simulink model "gm_wlanhdlTimeAndFrequencySynchronization"  (R2025a)
settings: Solver=FixedStepDiscrete  StartTime=0.0  StopTime=stopTime  RelTol=1e-3
InitFcn:
  | wlanFrontEndInit;
undefined symbols (not defined in the file or in its folder): a, b, c, Hd, wlanConfig
libraries: simulink x95, hdlsllib x16, hdlmdlgenlib x12, dspsrcs4 x3, dspsigops x3, dsphdlsigops2 x2, dsphdlfiltering2 x2
(part 6 of 11)

== system gm_wlanhdlTimeAndFrequencySynchronization/WLANTimeAndFrequencySynchronization/Coarse CFO Estimation and Correction/Coarse CFO Estimation/Iteration2 ==
  xin : Inport  OutDataTypeStr=fixdt(1, 32, 19)  SampleTime=6.25e-09
  yin : Inport  Port=2  OutDataTypeStr=fixdt(1, 32, 19)  SampleTime=6.25e-09
  zin : Inport  Port=3  OutDataTypeStr=fixdt(1, 34, 33)  SampleTime=6.25e-09
  lut_value : Inport  Port=4  OutDataTypeStr=fixdt(0, 31, 33)  SampleTime=6.25e-09
  idx : Inport  Port=5  OutDataTypeStr=fixdt(0, 6, 0)  SampleTime=6.25e-09
  MuxX : Switch  Criteria=u2 ~= 0  Threshold="fi(0,0,1,0,\"hex\",\"0\")"  OutDataTypeStr=fixdt(1, 32, 19)  SampleTime=6.25e-09  SaturateOnIntegerOverflow=off  InputSameDT=off
  MuxY : Switch  Criteria=u2 ~= 0  Threshold="fi(0,0,1,0,\"hex\",\"0\")"  OutDataTypeStr=fixdt(1, 32, 19)  SampleTime=6.25e-09  SaturateOnIntegerOverflow=off  InputSameDT=off
  MuxZ : Switch  Criteria=u2 ~= 0  Threshold="fi(0,0,1,0,\"hex\",\"0\")"  OutDataTypeStr=fixdt(1, 34, 33)  SampleTime=6.25e-09  SaturateOnIntegerOverflow=off  InputSameDT=off
  XAdder : Sum  OutDataTypeStr=fixdt(1, 32, 19)  SampleTime=6.25e-09
  XSubtractor : Sum  Inputs=+-  OutDataTypeStr=fixdt(1, 32, 19)  AccumDataTypeStr=fixdt(1, 32, 19)  SampleTime=6.25e-09
  YAdder : Sum  OutDataTypeStr=fixdt(1, 32, 19)  SampleTime=6.25e-09
  YSub : Sum  Inputs=+-  OutDataTypeStr=fixdt(1, 32, 19)  AccumDataTypeStr=fixdt(1, 32, 19)  SampleTime=6.25e-09
  ZAdder : Sum  OutDataTypeStr=fixdt(1, 34, 33)  SampleTime=6.25e-09
  ZSub : Sum  Inputs=+-  OutDataTypeStr=fixdt(1, 34, 33)  AccumDataTypeStr=fixdt(1, 34, 33)  SampleTime=6.25e-09
  compare : simulink/Logic and Bit Operations/Compare To Constant  relop=<  const=double(0)  OutDataTypeStr=boolean
  dynamic_shift : ArithShift  BitShiftNumberSource=Input port  BitShiftDirection=Right
      settings: InputPortMap=u0,p1
  dynamic_shift1 : ArithShift  BitShiftNumberSource=Input port  BitShiftDirection=Right
      settings: InputPortMap=u0,p1
  rd_{0..9} (10 alike) : Delay  DelayLength=double(1)  InitialCondition=0  SampleTime=6.25e-09
  xout : Outport  OutDataTypeStr=fixdt(1, 32, 19)  SampleTime=6.25e-09
  yout : Outport  Port=2  OutDataTypeStr=fixdt(1, 32, 19)  SampleTime=6.25e-09
  zout : Outport  Port=3  OutDataTypeStr=fixdt(1, 34, 33)  SampleTime=6.25e-09
  wires:
  MuxZ/1 -> zout/1
  rd_6/1 -> MuxY/3
  rd_9/1 -> MuxZ/3
  rd_2/1 -> MuxX/1
  rd_5/1 -> MuxY/1
  YSub/1 -> rd_6/1
  ZSub/1 -> rd_8/1
  xin/1 -> rd_0/1
  YAdder/1 -> rd_5/1
  lut_value/1 -> ZAdder/2, ZSub/2
  yin/1 -> rd_1/1
  rd_0/1 -> dynamic_shift/1, XAdder/1, XSubtractor/1
  MuxX/1 -> xout/1
  zin/1 -> rd_7/1
  MuxY/1 -> yout/1
  rd_1/1 -> compare/1, dynamic_shift1/1, YAdder/1, YSub/1
  idx/1 -> dynamic_shift1/2, dynamic_shift/2
  dynamic_shift1/1 -> XAdder/2, XSubtractor/2
  rd_3/1 -> MuxX/2, MuxY/2, MuxZ/2
  rd_7/1 -> ZSub/1, ZAdder/1
  rd_4/1 -> MuxX/3
  XAdder/1 -> rd_4/1
  compare/1 -> rd_3/1
  rd_8/1 -> MuxZ/1
  dynamic_shift/1 -> YSub/2, YAdder/2
  ZAdder/1 -> rd_9/1
  XSubtractor/1 -> rd_2/1

== system gm_wlanhdlTimeAndFrequencySynchronization/WLANTimeAndFrequencySynchronization/Coarse CFO Estimation and Correction/Coarse CFO Estimation/Iteration20 ==
  xin : Inport  OutDataTypeStr=fixdt(1, 32, 19)  SampleTime=6.25e-09
  yin : Inport  Port=2  OutDataTypeStr=fixdt(1, 32, 19)  SampleTime=6.25e-09
  zin : Inport  Port=3  OutDataTypeStr=fixdt(1, 34, 33)  SampleTime=6.25e-09
  lut_value : Inport  Port=4  OutDataTypeStr=fixdt(0, 31, 33)  SampleTime=6.25e-09
  idx : Inport  Port=5  OutDataTypeStr=fixdt(0, 6, 0)  SampleTime=6.25e-09
  MuxX : Switch  Criteria=u2 ~= 0  Threshold="fi(0,0,1,0,\"hex\",\"0\")"  OutDataTypeStr=fixdt(1, 32, 19)  SampleTime=6.25e-09  SaturateOnIntegerOverflow=off  InputSameDT=off
  MuxY : Switch  Criteria=u2 ~= 0  Threshold="fi(0,0,1,0,\"hex\",\"0\")"  OutDataTypeStr=fixdt(1, 32, 19)  SampleTime=6.25e-09  SaturateOnIntegerOverflow=off  InputSameDT=off
  MuxZ : Switch  Criteria=u2 ~= 0  Threshold="fi(0,0,1,0,\"hex\",\"0\")"  OutDataTypeStr=fixdt(1, 34, 33)  SampleTime=6.25e-09  SaturateOnIntegerOverflow=off  InputSameDT=off
  XAdder : Sum  OutDataTypeStr=fixdt(1, 32, 19)  SampleTime=6.25e-09
  XSubtractor : Sum  Inputs=+-  OutDataTypeStr=fixdt(1, 32, 19)  AccumDataTypeStr=fixdt(1, 32, 19)  SampleTime=6.25e-09
  YAdder : Sum  OutDataTypeStr=fixdt(1, 32, 19)  SampleTime=6.25e-09
  YSub : Sum  Inputs=+-  OutDataTypeStr=fixdt(1, 32, 19)  AccumDataTypeStr=fixdt(1, 32, 19)  SampleTime=6.25e-09
  ZAdder : Sum  OutDataTypeStr=fixdt(1, 34, 33)  SampleTime=6.25e-09
  ZSub : Sum  Inputs=+-  OutDataTypeStr=fixdt(1, 34, 33)  AccumDataTypeStr=fixdt(1, 34, 33)  SampleTime=6.25e-09
  compare : simulink/Logic and Bit Operations/Compare To Constant  relop=<  const=double(0)  OutDataTypeStr=boolean
  dynamic_shift : ArithShift  BitShiftNumberSource=Input port  BitShiftDirection=Right
      settings: InputPortMap=u0,p1
  dynamic_shift1 : ArithShift  BitShiftNumberSource=Input port  BitShiftDirection=Right
      settings: InputPortMap=u0,p1
  rd_{0..9} (10 alike) : Delay  DelayLength=double(1)  InitialCondition=0  SampleTime=6.25e-09
  xout : Outport  OutDataTypeStr=fixdt(1, 32, 19)  SampleTime=6.25e-09
  yout : Outport  Port=2  OutDataTypeStr=fixdt(1, 32, 19)  SampleTime=6.25e-09
  zout : Outport  Port=3  OutDataTypeStr=fixdt(1, 34, 33)  SampleTime=6.25e-09
  wires:
  MuxY/1 -> yout/1
  rd_4/1 -> MuxX/3
  rd_9/1 -> MuxZ/3
  rd_6/1 -> MuxY/3
  XAdder/1 -> rd_4/1
  ZAdder/1 -> rd_9/1
  rd_3/1 -> MuxX/2, MuxY/2, MuxZ/2
  yin/1 -> rd_1/1
  rd_8/1 -> MuxZ/1
  xin/1 -> rd_0/1
  MuxX/1 -> xout/1
  ZSub/1 -> rd_8/1
  zin/1 -> rd_7/1
  MuxZ/1 -> zout/1
  idx/1 -> dynamic_shift1/2, dynamic_shift/2
  rd_0/1 -> dynamic_shift/1, XSubtractor/1, XAdder/1
  rd_1/1 -> compare/1, dynamic_shift1/1, YAdder/1, YSub/1
  YSub/1 -> rd_6/1
  rd_2/1 -> MuxX/1
  dynamic_shift/1 -> YSub/2, YAdder/2
  XSubtractor/1 -> rd_2/1
  rd_7/1 -> ZSub/1, ZAdder/1
  rd_5/1 -> MuxY/1
  lut_value/1 -> ZAdder/2, ZSub/2
  dynamic_shift1/1 -> XAdder/2, XSubtractor/2
  compare/1 -> rd_3/1
  YAdder/1 -> rd_5/1

== system gm_wlanhdlTimeAndFrequencySynchronization/WLANTimeAndFrequencySynchronization/Coarse CFO Estimation and Correction/Coarse CFO Estimation/Iteration21 ==
  xin : Inport  OutDataTypeStr=fixdt(1, 32, 19)  SampleTime=6.25e-09
  yin : Inport  Port=2  OutDataTypeStr=fixdt(1, 32, 19)  SampleTime=6.25e-09
  zin : Inport  Port=3  OutDataTypeStr=fixdt(1, 34, 33)  SampleTime=6.25e-09
  lut_value : Inport  Port=4  OutDataTypeStr=fixdt(0, 31, 33)  SampleTime=6.25e-09
  idx : Inport  Port=5  OutDataTypeStr=fixdt(0, 6, 0)  SampleTime=6.25e-09
  MuxX : Switch  Criteria=u2 ~= 0  Threshold="fi(0,0,1,0,\"hex\",\"0\")"  OutDataTypeStr=fixdt(1, 32, 19)  SampleTime=6.25e-09  SaturateOnIntegerOverflow=off  InputSameDT=off
  MuxY : Switch  Criteria=u2 ~= 0  Threshold="fi(0,0,1,0,\"hex\",\"0\")"  OutDataTypeStr=fixdt(1, 32, 19)  SampleTime=6.25e-09  SaturateOnIntegerOverflow=off  InputSameDT=off
  MuxZ : Switch  Criteria=u2 ~= 0  Threshold="fi(0,0,1,0,\"hex\",\"0\")"  OutDataTypeStr=fixdt(1, 34, 33)  SampleTime=6.25e-09  SaturateOnIntegerOverflow=off  InputSameDT=off
  XAdder : Sum  OutDataTypeStr=fixdt(1, 32, 19)  SampleTime=6.25e-09
  XSubtractor : Sum  Inputs=+-  OutDataTypeStr=fixdt(1, 32, 19)  AccumDataTypeStr=fixdt(1, 32, 19)  SampleTime=6.25e-09
  YAdder : Sum  OutDataTypeStr=fixdt(1, 32, 19)  SampleTime=6.25e-09
  YSub : Sum  Inputs=+-  OutDataTypeStr=fixdt(1, 32, 19)  AccumDataTypeStr=fixdt(1, 32, 19)  SampleTime=6.25e-09
  ZAdder : Sum  OutDataTypeStr=fixdt(1, 34, 33)  SampleTime=6.25e-09
  ZSub : Sum  Inputs=+-  OutDataTypeStr=fixdt(1, 34, 33)  AccumDataTypeStr=fixdt(1, 34, 33)  SampleTime=6.25e-09
  compare : simulink/Logic and Bit Operations/Compare To Constant  relop=<  const=double(0)  OutDataTypeStr=boolean
  dynamic_shift : ArithShift  BitShiftNumberSource=Input port  BitShiftDirection=Right
      settings: InputPortMap=u0,p1
  dynamic_shift1 : ArithShift  BitShiftNumberSource=Input port  BitShiftDirection=Right
      settings: InputPortMap=u0,p1
  rd_{0..9} (10 alike) : Delay  DelayLength=double(1)  InitialCondition=0  SampleTime=6.25e-09
  xout : Outport  OutDataTypeStr=fixdt(1, 32, 19)  SampleTime=6.25e-09
  yout : Outport  Port=2  OutDataTypeStr=fixdt(1, 32, 19)  SampleTime=6.25e-09
  zout : Outport  Port=3  OutDataTypeStr=fixdt(1, 34, 33)  SampleTime=6.25e-09
  wires:
  MuxY/1 -> yout/1
  rd_2/1 -> MuxX/1
  rd_5/1 -> MuxY/1
  XAdder/1 -> rd_4/1
  MuxX/1 -> xout/1
  XSubtractor/1 -> rd_2/1
  rd_4/1 -> MuxX/3
  rd_8/1 -> MuxZ/1
  ZAdder/1 -> rd_9/1
  rd_3/1 -> MuxX/2, MuxY/2, MuxZ/2
  ZSub/1 -> rd_8/1
  yin/1 -> rd_1/1
  xin/1 -> rd_0/1
  rd_1/1 -> compare/1, dynamic_shift1/1, YAdder/1, YSub/1
  YAdder/1 -> rd_5/1
  dynamic_shift/1 -> YAdder/2, YSub/2
  MuxZ/1 -> zout/1
  rd_0/1 -> dynamic_shift/1, XAdder/1, XSubtractor/1
  idx/1 -> dynamic_shift/2, dynamic_shift1/2
  dynamic_shift1/1 -> XSubtractor/2, XAdder/2
  rd_6/1 -> MuxY/3
  rd_7/1 -> ZSub/1, ZAdder/1
  lut_value/1 -> ZSub/2, ZAdder/2
  compare/1 -> rd_3/1
  rd_9/1 -> MuxZ/3
  zin/1 -> rd_7/1
  YSub/1 -> rd_6/1

== system gm_wlanhdlTimeAndFrequencySynchronization/WLANTimeAndFrequencySynchronization/Coarse CFO Estimation and Correction/Coarse CFO Estimation/Iteration22 ==
  xin : Inport  OutDataTypeStr=fixdt(1, 32, 19)  SampleTime=6.25e-09
  yin : Inport  Port=2  OutDataTypeStr=fixdt(1, 32, 19)  SampleTime=6.25e-09
  zin : Inport  Port=3  OutDataTypeStr=fixdt(1, 34, 33)  SampleTime=6.25e-09
  lut_value : Inport  Port=4  OutDataTypeStr=fixdt(0, 31, 33)  SampleTime=6.25e-09
  idx : Inport  Port=5  OutDataTypeStr=fixdt(0, 6, 0)  SampleTime=6.25e-09
  MuxX : Switch  Criteria=u2 ~= 0  Threshold="fi(0,0,1,0,\"hex\",\"0\")"  OutDataTypeStr=fixdt(1, 32, 19)  SampleTime=6.25e-09  SaturateOnIntegerOverflow=off  InputSameDT=off
  MuxY : Switch  Criteria=u2 ~= 0  Threshold="fi(0,0,1,0,\"hex\",\"0\")"  OutDataTypeStr=fixdt(1, 32, 19)  SampleTime=6.25e-09  SaturateOnIntegerOverflow=off  InputSameDT=off
  MuxZ : Switch  Criteria=u2 ~= 0  Threshold="fi(0,0,1,0,\"hex\",\"0\")"  OutDataTypeStr=fixdt(1, 34, 33)  SampleTime=6.25e-09  SaturateOnIntegerOverflow=off  InputSameDT=off
  XAdder : Sum  OutDataTypeStr=fixdt(1, 32, 19)  SampleTime=6.25e-09
  XSubtractor : Sum  Inputs=+-  OutDataTypeStr=fixdt(1, 32, 19)  AccumDataTypeStr=fixdt(1, 32, 19)  SampleTime=6.25e-09
  YAdder : Sum  OutDataTypeStr=fixdt(1, 32, 19)  SampleTime=6.25e-09
  YSub : Sum  Inputs=+-  OutDataTypeStr=fixdt(1, 32, 19)  AccumDataTypeStr=fixdt(1, 32, 19)  SampleTime=6.25e-09
  ZAdder : Sum  OutDataTypeStr=fixdt(1, 34, 33)  SampleTime=6.25e-09
  ZSub : Sum  Inputs=+-  OutDataTypeStr=fixdt(1, 34, 33)  AccumDataTypeStr=fixdt(1, 34, 33)  SampleTime=6.25e-09
  compare : simulink/Logic and Bit Operations/Compare To Constant  relop=<  const=double(0)  OutDataTypeStr=boolean
  dynamic_shift : ArithShift  BitShiftNumberSource=Input port  BitShiftDirection=Right
      settings: InputPortMap=u0,p1
  dynamic_shift1 : ArithShift  BitShiftNumberSource=Input port  BitShiftDirection=Right
      settings: InputPortMap=u0,p1
  rd_{0..9} (10 alike) : Delay  DelayLength=double(1)  InitialCondition=0  SampleTime=6.25e-09
  xout : Outport  OutDataTypeStr=fixdt(1, 32, 19)  SampleTime=6.25e-09
  yout : Outport  Port=2  OutDataTypeStr=fixdt(1, 32, 19)  SampleTime=6.25e-09
  zout : Outport  Port=3  OutDataTypeStr=fixdt(1, 34, 33)  SampleTime=6.25e-09
  wires:
  MuxX/1 -> xout/1
  MuxY/1 -> yout/1
  rd_4/1 -> MuxX/3
  rd_2/1 -> MuxX/1
  rd_3/1 -> MuxX/2, MuxY/2, MuxZ/2
  XAdder/1 -> rd_4/1
  XSubtractor/1 -> rd_2/1
  ZAdder/1 -> rd_9/1
  rd_9/1 -> MuxZ/3
  ZSub/1 -> rd_8/1
  compare/1 -> rd_3/1
  rd_8/1 -> MuxZ/1
  rd_5/1 -> MuxY/1
  yin/1 -> rd_1/1
  rd_1/1 -> compare/1, dynamic_shift1/1, YAdder/1, YSub/1
  dynamic_shift1/1 -> XAdder/2, XSubtractor/2
  zin/1 -> rd_7/1
  MuxZ/1 -> zout/1
  idx/1 -> dynamic_shift1/2, dynamic_shift/2
  YSub/1 -> rd_6/1
  rd_0/1 -> dynamic_shift/1, XSubtractor/1, XAdder/1
  dynamic_shift/1 -> YSub/2, YAdder/2
  rd_7/1 -> ZSub/1, ZAdder/1
  rd_6/1 -> MuxY/3
  lut_value/1 -> ZAdder/2, ZSub/2
  xin/1 -> rd_0/1
  YAdder/1 -> rd_5/1

== system gm_wlanhdlTimeAndFrequencySynchronization/WLANTimeAndFrequencySynchronization/Coarse CFO Estimation and Correction/Coarse CFO Estimation/Iteration23 ==
  xin : Inport  OutDataTypeStr=fixdt(1, 32, 19)  SampleTime=6.25e-09
  yin : Inport  Port=2  OutDataTypeStr=fixdt(1, 32, 19)  SampleTime=6.25e-09
  zin : Inport  Port=3  OutDataTypeStr=fixdt(1, 34, 33)  SampleTime=6.25e-09
  lut_value : Inport  Port=4  OutDataTypeStr=fixdt(0, 31, 33)  SampleTime=6.25e-09
  idx : Inport  Port=5  OutDataTypeStr=fixdt(0, 6, 0)  SampleTime=6.25e-09
  MuxX : Switch  Criteria=u2 ~= 0  Threshold="fi(0,0,1,0,\"hex\",\"0\")"  OutDataTypeStr=fixdt(1, 32, 19)  SampleTime=6.25e-09  SaturateOnIntegerOverflow=off  InputSameDT=off
  MuxY : Switch  Criteria=u2 ~= 0  Threshold="fi(0,0,1,0,\"hex\",\"0\")"  OutDataTypeStr=fixdt(1, 32, 19)  SampleTime=6.25e-09  SaturateOnIntegerOverflow=off  InputSameDT=off
  MuxZ : Switch  Criteria=u2 ~= 0  Threshold="fi(0,0,1,0,\"hex\",\"0\")"  OutDataTypeStr=fixdt(1, 34, 33)  SampleTime=6.25e-09  SaturateOnIntegerOverflow=off  InputSameDT=off
  XAdder : Sum  OutDataTypeStr=fixdt(1, 32, 19)  SampleTime=6.25e-09
  XSubtractor : Sum  Inputs=+-  OutDataTypeStr=fixdt(1, 32, 19)  AccumDataTypeStr=fixdt(1, 32, 19)  SampleTime=6.25e-09
  YAdder : Sum  OutDataTypeStr=fixdt(1, 32, 19)  SampleTime=6.25e-09
  YSub : Sum  Inputs=+-  OutDataTypeStr=fixdt(1, 32, 19)  AccumDataTypeStr=fixdt(1, 32, 19)  SampleTime=6.25e-09
  ZAdder : Sum  OutDataTypeStr=fixdt(1, 34, 33)  SampleTime=6.25e-09
  ZSub : Sum  Inputs=+-  OutDataTypeStr=fixdt(1, 34, 33)  AccumDataTypeStr=fixdt(1, 34, 33)  SampleTime=6.25e-09
  compare : simulink/Logic and Bit Operations/Compare To Constant  relop=<  const=double(0)  OutDataTypeStr=boolean
  dynamic_shift : ArithShift  BitShiftNumberSource=Input port  BitShiftDirection=Right
      settings: InputPortMap=u0,p1
  dynamic_shift1 : ArithShift  BitShiftNumberSource=Input port  BitShiftDirection=Right
      settings: InputPortMap=u0,p1
  rd_{0..9} (10 alike) : Delay  DelayLength=double(1)  InitialCondition=0  SampleTime=6.25e-09
  xout : Outport  OutDataTypeStr=fixdt(1, 32, 19)  SampleTime=6.25e-09
  yout : Outport  Port=2  OutDataTypeStr=fixdt(1, 32, 19)  SampleTime=6.25e-09
  zout : Outport  Port=3  OutDataTypeStr=fixdt(1, 34, 33)  SampleTime=6.25e-09
  wires:
  MuxZ/1 -> zout/1
  rd_3/1 -> MuxX/2, MuxZ/2, MuxY/2
  rd_9/1 -> MuxZ/3
  YAdder/1 -> rd_5/1
  yin/1 -> rd_1/1
  MuxX/1 -> xout/1
  XSubtractor/1 -> rd_2/1
  rd_1/1 -> compare/1, dynamic_shift1/1, YAdder/1, YSub/1
  rd_5/1 -> MuxY/1
  ZSub/1 -> rd_8/1
  MuxY/1 -> yout/1
  XAdder/1 -> rd_4/1
  xin/1 -> rd_0/1
  idx/1 -> dynamic_shift/2, dynamic_shift1/2
  rd_0/1 -> dynamic_shift/1, XAdder/1, XSubtractor/1
  dynamic_shift1/1 -> XSubtractor/2, XAdder/2
  zin/1 -> rd_7/1
  ZAdder/1 -> rd_9/1
  rd_4/1 -> MuxX/3
  rd_6/1 -> MuxY/3
  YSub/1 -> rd_6/1
  rd_7/1 -> ZSub/1, ZAdder/1
  rd_2/1 -> MuxX/1
  dynamic_shift/1 -> YAdder/2, YSub/2
  rd_8/1 -> MuxZ/1
  lut_value/1 -> ZSub/2, ZAdder/2
  compare/1 -> rd_3/1

== system gm_wlanhdlTimeAndFrequencySynchronization/WLANTimeAndFrequencySynchronization/Coarse CFO Estimation and Correction/Coarse CFO Estimation/Iteration24 ==
  xin : Inport  OutDataTypeStr=fixdt(1, 32, 19)  SampleTime=6.25e-09
  yin : Inport  Port=2  OutDataTypeStr=fixdt(1, 32, 19)  SampleTime=6.25e-09
  zin : Inport  Port=3  OutDataTypeStr=fixdt(1, 34, 33)  SampleTime=6.25e-09
  lut_value : Inport  Port=4  OutDataTypeStr=fixdt(0, 31, 33)  SampleTime=6.25e-09
  idx : Inport  Port=5  OutDataTypeStr=fixdt(0, 6, 0)  SampleTime=6.25e-09
  MuxX : Switch  Criteria=u2 ~= 0  Threshold="fi(0,0,1,0,\"hex\",\"0\")"  OutDataTypeStr=fixdt(1, 32, 19)  SampleTime=6.25e-09  SaturateOnIntegerOverflow=off  InputSameDT=off
  MuxY : Switch  Criteria=u2 ~= 0  Threshold="fi(0,0,1,0,\"hex\",\"0\")"  OutDataTypeStr=fixdt(1, 32, 19)  SampleTime=6.25e-09  SaturateOnIntegerOverflow=off  InputSameDT=off
  MuxZ : Switch  Criteria=u2 ~= 0  Threshold="fi(0,0,1,0,\"hex\",\"0\")"  OutDataTypeStr=fixdt(1, 34, 33)  SampleTime=6.25e-09  SaturateOnIntegerOverflow=off  InputSameDT=off
  XAdder : Sum  OutDataTypeStr=fixdt(1, 32, 19)  SampleTime=6.25e-09
  XSubtractor : Sum  Inputs=+-  OutDataTypeStr=fixdt(1, 32, 19)  AccumDataTypeStr=fixdt(1, 32, 19)  SampleTime=6.25e-09
  YAdder : Sum  OutDataTypeStr=fixdt(1, 32, 19)  SampleTime=6.25e-09
  YSub : Sum  Inputs=+-  OutDataTypeStr=fixdt(1, 32, 19)  AccumDataTypeStr=fixdt(1, 32, 19)  SampleTime=6.25e-09
  ZAdder : Sum  OutDataTypeStr=fixdt(1, 34, 33)  SampleTime=6.25e-09
  ZSub : Sum  Inputs=+-  OutDataTypeStr=fixdt(1, 34, 33)  AccumDataTypeStr=fixdt(1, 34, 33)  SampleTime=6.25e-09
  compare : simulink/Logic and Bit Operations/Compare To Constant  relop=<  const=double(0)  OutDataTypeStr=boolean
  dynamic_shift : ArithShift  BitShiftNumberSource=Input port  BitShiftDirection=Right
      settings: InputPortMap=u0,p1
  dynamic_shift1 : ArithShift  BitShiftNumberSource=Input port  BitShiftDirection=Right
      settings: InputPortMap=u0,p1
  rd_{0..9} (10 alike) : Delay  DelayLength=double(1)  InitialCondition=0  SampleTime=6.25e-09
  xout : Outport  OutDataTypeStr=fixdt(1, 32, 19)  SampleTime=6.25e-09
  yout : Outport  Port=2  OutDataTypeStr=fixdt(1, 32, 19)  SampleTime=6.25e-09
  zout : Outport  Port=3  OutDataTypeStr=fixdt(1, 34, 33)  SampleTime=6.25e-09
  wires:
  MuxZ/1 -> zout/1
  rd_2/1 -> MuxX/1
  rd_9/1 -> MuxZ/3
  rd_3/1 -> MuxX/2, MuxY/2, MuxZ/2
  rd_6/1 -> MuxY/3
  MuxY/1 -> yout/1
  rd_8/1 -> MuxZ/1
  XAdder/1 -> rd_4/1
  ZAdder/1 -> rd_9/1
  yin/1 -> rd_1/1
  MuxX/1 -> xout/1
  compare/1 -> rd_3/1
  rd_5/1 -> MuxY/1
  xin/1 -> rd_0/1
  rd_7/1 -> ZSub/1, ZAdder/1
  rd_1/1 -> compare/1, YAdder/1, dynamic_shift1/1, YSub/1
  zin/1 -> rd_7/1
  YSub/1 -> rd_6/1
  idx/1 -> dynamic_shift1/2, dynamic_shift/2
  rd_0/1 -> dynamic_shift/1, XSubtractor/1, XAdder/1
  dynamic_shift/1 -> YSub/2, YAdder/2
  ZSub/1 -> rd_8/1
  dynamic_shift1/1 -> XAdder/2, XSubtractor/2
  rd_4/1 -> MuxX/3
  lut_value/1 -> ZAdder/2, ZSub/2
  XSubtractor/1 -> rd_2/1
  YAdder/1 -> rd_5/1

== system gm_wlanhdlTimeAndFrequencySynchronization/WLANTimeAndFrequencySynchronization/Coarse CFO Estimation and Correction/Coarse CFO Estimation/Iteration25 ==
  xin : Inport  OutDataTypeStr=fixdt(1, 32, 19)  SampleTime=6.25e-09
  yin : Inport  Port=2  OutDataTypeStr=fixdt(1, 32, 19)  SampleTime=6.25e-09
  zin : Inport  Port=3  OutDataTypeStr=fixdt(1, 34, 33)  SampleTime=6.25e-09
  lut_value : Inport  Port=4  OutDataTypeStr=fixdt(0, 31, 33)  SampleTime=6.25e-09
  idx : Inport  Port=5  OutDataTypeStr=fixdt(0, 6, 0)  SampleTime=6.25e-09
  MuxX : Switch  Criteria=u2 ~= 0  Threshold="fi(0,0,1,0,\"hex\",\"0\")"  OutDataTypeStr=fixdt(1, 32, 19)  SampleTime=6.25e-09  SaturateOnIntegerOverflow=off  InputSameDT=off
  MuxY : Switch  Criteria=u2 ~= 0  Threshold="fi(0,0,1,0,\"hex\",\"0\")"  OutDataTypeStr=fixdt(1, 32, 19)  SampleTime=6.25e-09  SaturateOnIntegerOverflow=off  InputSameDT=off
  MuxZ : Switch  Criteria=u2 ~= 0  Threshold="fi(0,0,1,0,\"hex\",\"0\")"  OutDataTypeStr=fixdt(1, 34, 33)  SampleTime=6.25e-09  SaturateOnIntegerOverflow=off  InputSameDT=off
  XAdder : Sum  OutDataTypeStr=fixdt(1, 32, 19)  SampleTime=6.25e-09
  XSubtractor : Sum  Inputs=+-  OutDataTypeStr=fixdt(1, 32, 19)  AccumDataTypeStr=fixdt(1, 32, 19)  SampleTime=6.25e-09
  YAdder : Sum  OutDataTypeStr=fixdt(1, 32, 19)  SampleTime=6.25e-09
  YSub : Sum  Inputs=+-  OutDataTypeStr=fixdt(1, 32, 19)  AccumDataTypeStr=fixdt(1, 32, 19)  SampleTime=6.25e-09
  ZAdder : Sum  OutDataTypeStr=fixdt(1, 34, 33)  SampleTime=6.25e-09
  ZSub : Sum  Inputs=+-  OutDataTypeStr=fixdt(1, 34, 33)  AccumDataTypeStr=fixdt(1, 34, 33)  SampleTime=6.25e-09
  compare : simulink/Logic and Bit Operations/Compare To Constant  relop=<  const=double(0)  OutDataTypeStr=boolean
  dynamic_shift : ArithShift  BitShiftNumberSource=Input port  BitShiftDirection=Right
      settings: InputPortMap=u0,p1
  dynamic_shift1 : ArithShift  BitShiftNumberSource=Input port  BitShiftDirection=Right
      settings: InputPortMap=u0,p1
  rd_{0..9} (10 alike) : Delay  DelayLength=double(1)  InitialCondition=0  SampleTime=6.25e-09
  xout : Outport  OutDataTypeStr=fixdt(1, 32, 19)  SampleTime=6.25e-09
  yout : Outport  Port=2  OutDataTypeStr=fixdt(1, 32, 19)  SampleTime=6.25e-09
  zout : Outport  Port=3  OutDataTypeStr=fixdt(1, 34, 33)  SampleTime=6.25e-09
  wires:
  MuxZ/1 -> zout/1
  rd_2/1 -> MuxX/1
  rd_4/1 -> MuxX/3
  rd_9/1 -> MuxZ/3
  rd_3/1 -> MuxX/2, MuxY/2, MuxZ/2
  rd_8/1 -> MuxZ/1
  rd_6/1 -> MuxY/3
  MuxY/1 -> yout/1
  rd_5/1 -> MuxY/1
  XSubtractor/1 -> rd_2/1
  ZAdder/1 -> rd_9/1
  ZSub/1 -> rd_8/1
  lut_value/1 -> ZSub/2, ZAdder/2
  xin/1 -> rd_0/1
  YAdder/1 -> rd_5/1
  XAdder/1 -> rd_4/1
  rd_1/1 -> compare/1, dynamic_shift1/1, YAdder/1, YSub/1
  yin/1 -> rd_1/1
  zin/1 -> rd_7/1
  idx/1 -> dynamic_shift/2, dynamic_shift1/2
  MuxX/1 -> xout/1
  dynamic_shift/1 -> YAdder/2, YSub/2
  compare/1 -> rd_3/1
  rd_0/1 -> dynamic_shift/1, XSubtractor/1, XAdder/1
  dynamic_shift1/1 -> XSubtractor/2, XAdder/2
  rd_7/1 -> ZSub/1, ZAdder/1
  YSub/1 -> rd_6/1

== system gm_wlanhdlTimeAndFrequencySynchronization/WLANTimeAndFrequencySynchronization/Coarse CFO Estimation and Correction/Coarse CFO Estimation/Iteration26 ==
  xin : Inport  OutDataTypeStr=fixdt(1, 32, 19)  SampleTime=6.25e-09
  yin : Inport  Port=2  OutDataTypeStr=fixdt(1, 32, 19)  SampleTime=6.25e-09
  zin : Inport  Port=3  OutDataTypeStr=fixdt(1, 34, 33)  SampleTime=6.25e-09
  lut_value : Inport  Port=4  OutDataTypeStr=fixdt(0, 31, 33)  SampleTime=6.25e-09
  idx : Inport  Port=5  OutDataTypeStr=fixdt(0, 6, 0)  SampleTime=6.25e-09
  MuxX : Switch  Criteria=u2 ~= 0  Threshold="fi(0,0,1,0,\"hex\",\"0\")"  OutDataTypeStr=fixdt(1, 32, 19)  SampleTime=6.25e-09  SaturateOnIntegerOverflow=off  InputSameDT=off
  MuxY : Switch  Criteria=u2 ~= 0  Threshold="fi(0,0,1,0,\"hex\",\"0\")"  OutDataTypeStr=fixdt(1, 32, 19)  SampleTime=6.25e-09  SaturateOnIntegerOverflow=off  InputSameDT=off
  MuxZ : Switch  Criteria=u2 ~= 0  Threshold="fi(0,0,1,0,\"hex\",\"0\")"  OutDataTypeStr=fixdt(1, 34, 33)  SampleTime=6.25e-09  SaturateOnIntegerOverflow=off  InputSameDT=off
  XAdder : Sum  OutDataTypeStr=fixdt(1, 32, 19)  SampleTime=6.25e-09
  XSubtractor : Sum  Inputs=+-  OutDataTypeStr=fixdt(1, 32, 19)  AccumDataTypeStr=fixdt(1, 32, 19)  SampleTime=6.25e-09
  YAdder : Sum  OutDataTypeStr=fixdt(1, 32, 19)  SampleTime=6.25e-09
  YSub : Sum  Inputs=+-  OutDataTypeStr=fixdt(1, 32, 19)  AccumDataTypeStr=fixdt(1, 32, 19)  SampleTime=6.25e-09
  ZAdder : Sum  OutDataTypeStr=fixdt(1, 34, 33)  SampleTime=6.25e-09
  ZSub : Sum  Inputs=+-  OutDataTypeStr=fixdt(1, 34, 33)  AccumDataTypeStr=fixdt(1, 34, 33)  SampleTime=6.25e-09
  compare : simulink/Logic and Bit Operations/Compare To Constant  relop=<  const=double(0)  OutDataTypeStr=boolean
  dynamic_shift : ArithShift  BitShiftNumberSource=Input port  BitShiftDirection=Right
      settings: InputPortMap=u0,p1
  dynamic_shift1 : ArithShift  BitShiftNumberSource=Input port  BitShiftDirection=Right
      settings: InputPortMap=u0,p1
  rd_{0..9} (10 alike) : Delay  DelayLength=double(1)  InitialCondition=0  SampleTime=6.25e-09
  xout : Outport  OutDataTypeStr=fixdt(1, 32, 19)  SampleTime=6.25e-09
  yout : Outport  Port=2  OutDataTypeStr=fixdt(1, 32, 19)  SampleTime=6.25e-09
  zout : Outport  Port=3  OutDataTypeStr=fixdt(1, 34, 33)  SampleTime=6.25e-09
  wires:
  MuxX/1 -> xout/1
  MuxY/1 -> yout/1
  rd_9/1 -> MuxZ/3
  rd_8/1 -> MuxZ/1
  ZAdder/1 -> rd_9/1
  ZSub/1 -> rd_8/1
  rd_6/1 -> MuxY/3
  rd_5/1 -> MuxY/1
  XAdder/1 -> rd_4/1
  XSubtractor/1 -> rd_2/1
  xin/1 -> rd_0/1
  rd_3/1 -> MuxX/2, MuxY/2, MuxZ/2
  rd_1/1 -> compare/1, dynamic_shift1/1, YAdder/1, YSub/1
  rd_0/1 -> dynamic_shift/1, XSubtractor/1, XAdder/1
  YSub/1 -> rd_6/1
  MuxZ/1 -> zout/1
  zin/1 -> rd_7/1
  rd_7/1 -> ZSub/1, ZAdder/1
  rd_4/1 -> MuxX/3
  YAdder/1 -> rd_5/1
  rd_2/1 -> MuxX/1
  dynamic_shift/1 -> YSub/2, YAdder/2
  yin/1 -> rd_1/1
  idx/1 -> dynamic_shift1/2, dynamic_shift/2
  compare/1 -> rd_3/1
  lut_value/1 -> ZAdder/2, ZSub/2
  dynamic_shift1/1 -> XAdder/2, XSubtractor/2

== system gm_wlanhdlTimeAndFrequencySynchronization/WLANTimeAndFrequencySynchronization/Coarse CFO Estimation and Correction/Coarse CFO Estimation/Iteration27 ==
  xin : Inport  OutDataTypeStr=fixdt(1, 32, 19)  SampleTime=6.25e-09
  yin : Inport  Port=2  OutDataTypeStr=fixdt(1, 32, 19)  SampleTime=6.25e-09
  zin : Inport  Port=3  OutDataTypeStr=fixdt(1, 34, 33)  SampleTime=6.25e-09
  lut_value : Inport  Port=4  OutDataTypeStr=fixdt(0, 31, 33)  SampleTime=6.25e-09
  idx : Inport  Port=5  OutDataTypeStr=fixdt(0, 6, 0)  SampleTime=6.25e-09
  MuxX : Switch  Criteria=u2 ~= 0  Threshold="fi(0,0,1,0,\"hex\",\"0\")"  OutDataTypeStr=fixdt(1, 32, 19)  SampleTime=6.25e-09  SaturateOnIntegerOverflow=off  InputSameDT=off
  MuxY : Switch  Criteria=u2 ~= 0  Threshold="fi(0,0,1,0,\"hex\",\"0\")"  OutDataTypeStr=fixdt(1, 32, 19)  SampleTime=6.25e-09  SaturateOnIntegerOverflow=off  InputSameDT=off
  MuxZ : Switch  Criteria=u2 ~= 0  Threshold="fi(0,0,1,0,\"hex\",\"0\")"  OutDataTypeStr=fixdt(1, 34, 33)  SampleTime=6.25e-09  SaturateOnIntegerOverflow=off  InputSameDT=off
  XAdder : Sum  OutDataTypeStr=fixdt(1, 32, 19)  SampleTime=6.25e-09
  XSubtractor : Sum  Inputs=+-  OutDataTypeStr=fixdt(1, 32, 19)  AccumDataTypeStr=fixdt(1, 32, 19)  SampleTime=6.25e-09
  YAdder : Sum  OutDataTypeStr=fixdt(1, 32, 19)  SampleTime=6.25e-09
  YSub : Sum  Inputs=+-  OutDataTypeStr=fixdt(1, 32, 19)  AccumDataTypeStr=fixdt(1, 32, 19)  SampleTime=6.25e-09
  ZAdder : Sum  OutDataTypeStr=fixdt(1, 34, 33)  SampleTime=6.25e-09
  ZSub : Sum  Inputs=+-  OutDataTypeStr=fixdt(1, 34, 33)  AccumDataTypeStr=fixdt(1, 34, 33)  SampleTime=6.25e-09
  compare : simulink/Logic and Bit Operations/Compare To Constant  relop=<  const=double(0)  OutDataTypeStr=boolean
  dynamic_shift : ArithShift  BitShiftNumberSource=Input port  BitShiftDirection=Right
      settings: InputPortMap=u0,p1
  dynamic_shift1 : ArithShift  BitShiftNumberSource=Input port  BitShiftDirection=Right
      settings: InputPortMap=u0,p1
  rd_{0..9} (10 alike) : Delay  DelayLength=double(1)  InitialCondition=0  SampleTime=6.25e-09
  xout : Outport  OutDataTypeStr=fixdt(1, 32, 19)  SampleTime=6.25e-09
  yout : Outport  Port=2  OutDataTypeStr=fixdt(1, 32, 19)  SampleTime=6.25e-09
  zout : Outport  Port=3  OutDataTypeStr=fixdt(1, 34, 33)  SampleTime=6.25e-09
  wires:
  MuxX/1 -> xout/1
  MuxY/1 -> yout/1
  rd_6/1 -> MuxY/3
  rd_3/1 -> MuxX/2, MuxZ/2, MuxY/2
  rd_8/1 -> MuxZ/1
  XAdder/1 -> rd_4/1
  MuxZ/1 -> zout/1
  YSub/1 -> rd_6/1
  YAdder/1 -> rd_5/1
  yin/1 -> rd_1/1
  rd_9/1 -> MuxZ/3
  ZAdder/1 -> rd_9/1
  xin/1 -> rd_0/1
  rd_7/1 -> ZSub/1, ZAdder/1
  lut_value/1 -> ZSub/2, ZAdder/2
  XSubtractor/1 -> rd_2/1
  rd_1/1 -> compare/1, YAdder/1, dynamic_shift1/1, YSub/1
  rd_2/1 -> MuxX/1
  rd_5/1 -> MuxY/1
  ZSub/1 -> rd_8/1
  rd_0/1 -> dynamic_shift/1, XSubtractor/1, XAdder/1
  idx/1 -> dynamic_shift/2, dynamic_shift1/2
  rd_4/1 -> MuxX/3
  compare/1 -> rd_3/1
  dynamic_shift/1 -> YAdder/2, YSub/2
  zin/1 -> rd_7/1
  dynamic_shift1/1 -> XSubtractor/2, XAdder/2

== system gm_wlanhdlTimeAndFrequencySynchronization/WLANTimeAndFrequencySynchronization/Coarse CFO Estimation and Correction/Coarse CFO Estimation/Iteration28 ==
  xin : Inport  OutDataTypeStr=fixdt(1, 32, 19)  SampleTime=6.25e-09
  yin : Inport  Port=2  OutDataTypeStr=fixdt(1, 32, 19)  SampleTime=6.25e-09
  zin : Inport  Port=3  OutDataTypeStr=fixdt(1, 34, 33)  SampleTime=6.25e-09
  lut_value : Inport  Port=4  OutDataTypeStr=fixdt(0, 31, 33)  SampleTime=6.25e-09
  idx : Inport  Port=5  OutDataTypeStr=fixdt(0, 6, 0)  SampleTime=6.25e-09
  MuxX : Switch  Criteria=u2 ~= 0  Threshold="fi(0,0,1,0,\"hex\",\"0\")"  OutDataTypeStr=fixdt(1, 32, 19)  SampleTime=6.25e-09  SaturateOnIntegerOverflow=off  InputSameDT=off
  MuxY : Switch  Criteria=u2 ~= 0  Threshold="fi(0,0,1,0,\"hex\",\"0\")"  OutDataTypeStr=fixdt(1, 32, 19)  SampleTime=6.25e-09  SaturateOnIntegerOverflow=off  InputSameDT=off
  MuxZ : Switch  Criteria=u2 ~= 0  Threshold="fi(0,0,1,0,\"hex\",\"0\")"  OutDataTypeStr=fixdt(1, 34, 33)  SampleTime=6.25e-09  SaturateOnIntegerOverflow=off  InputSameDT=off
  XAdder : Sum  OutDataTypeStr=fixdt(1, 32, 19)  SampleTime=6.25e-09
  XSubtractor : Sum  Inputs=+-  OutDataTypeStr=fixdt(1, 32, 19)  AccumDataTypeStr=fixdt(1, 32, 19)  SampleTime=6.25e-09
  YAdder : Sum  OutDataTypeStr=fixdt(1, 32, 19)  SampleTime=6.25e-09
  YSub : Sum  Inputs=+-  OutDataTypeStr=fixdt(1, 32, 19)  AccumDataTypeStr=fixdt(1, 32, 19)  SampleTime=6.25e-09
  ZAdder : Sum  OutDataTypeStr=fixdt(1, 34, 33)  SampleTime=6.25e-09
  ZSub : Sum  Inputs=+-  OutDataTypeStr=fixdt(1, 34, 33)  AccumDataTypeStr=fixdt(1, 34, 33)  SampleTime=6.25e-09
  compare : simulink/Logic and Bit Operations/Compare To Constant  relop=<  const=double(0)  OutDataTypeStr=boolean
  dynamic_shift : ArithShift  BitShiftNumberSource=Input port  BitShiftDirection=Right
      settings: InputPortMap=u0,p1
  dynamic_shift1 : ArithShift  BitShiftNumberSource=Input port  BitShiftDirection=Right
      settings: InputPortMap=u0,p1
  rd_{0..9} (10 alike) : Delay  DelayLength=double(1)  InitialCondition=0  SampleTime=6.25e-09
  xout : Outport  OutDataTypeStr=fixdt(1, 32, 19)  SampleTime=6.25e-09
  yout : Outport  Port=2  OutDataTypeStr=fixdt(1, 32, 19)  SampleTime=6.25e-09
  zout : Outport  Port=3  OutDataTypeStr=fixdt(1, 34, 33)  SampleTime=6.25e-09
  wires:
  MuxZ/1 -> zout/1
  rd_4/1 -> MuxX/3
  rd_5/1 -> MuxY/1
  XSubtractor/1 -> rd_2/1
  MuxY/1 -> yout/1
  rd_9/1 -> MuxZ/3
  ZSub/1 -> rd_8/1
  xin/1 -> rd_0/1
  MuxX/1 -> xout/1
  rd_1/1 -> compare/1, dynamic_shift1/1, YAdder/1, YSub/1
  YAdder/1 -> rd_5/1
  rd_8/1 -> MuxZ/1
  idx/1 -> dynamic_shift1/2, dynamic_shift/2
  XAdder/1 -> rd_4/1
  rd_0/1 -> dynamic_shift/1, XSubtractor/1, XAdder/1
  rd_6/1 -> MuxY/3
  yin/1 -> rd_1/1
  zin/1 -> rd_7/1
  rd_7/1 -> ZSub/1, ZAdder/1
  rd_2/1 -> MuxX/1
  dynamic_shift/1 -> YSub/2, YAdder/2
  dynamic_shift1/1 -> XAdder/2, XSubtractor/2
  ZAdder/1 -> rd_9/1
  compare/1 -> rd_3/1
  rd_3/1 -> MuxX/2, MuxY/2, MuxZ/2
  YSub/1 -> rd_6/1
  lut_value/1 -> ZAdder/2, ZSub/2

== system gm_wlanhdlTimeAndFrequencySynchronization/WLANTimeAndFrequencySynchronization/Coarse CFO Estimation and Correction/Coarse CFO Estimation/Iteration29 ==
  xin : Inport  OutDataTypeStr=fixdt(1, 32, 19)  SampleTime=6.25e-09
  yin : Inport  Port=2  OutDataTypeStr=fixdt(1, 32, 19)  SampleTime=6.25e-09
  zin : Inport  Port=3  OutDataTypeStr=fixdt(1, 34, 33)  SampleTime=6.25e-09
  lut_value : Inport  Port=4  OutDataTypeStr=fixdt(0, 31, 33)  SampleTime=6.25e-09
  idx : Inport  Port=5  OutDataTypeStr=fixdt(0, 6, 0)  SampleTime=6.25e-09
  MuxX : Switch  Criteria=u2 ~= 0  Threshold="fi(0,0,1,0,\"hex\",\"0\")"  OutDataTypeStr=fixdt(1, 32, 19)  SampleTime=6.25e-09  SaturateOnIntegerOverflow=off  InputSameDT=off
  MuxY : Switch  Criteria=u2 ~= 0  Threshold="fi(0,0,1,0,\"hex\",\"0\")"  OutDataTypeStr=fixdt(1, 32, 19)  SampleTime=6.25e-09  SaturateOnIntegerOverflow=off  InputSameDT=off
  MuxZ : Switch  Criteria=u2 ~= 0  Threshold="fi(0,0,1,0,\"hex\",\"0\")"  OutDataTypeStr=fixdt(1, 34, 33)  SampleTime=6.25e-09  SaturateOnIntegerOverflow=off  InputSameDT=off
  XAdder : Sum  OutDataTypeStr=fixdt(1, 32, 19)  SampleTime=6.25e-09
  XSubtractor : Sum  Inputs=+-  OutDataTypeStr=fixdt(1, 32, 19)  AccumDataTypeStr=fixdt(1, 32, 19)  SampleTime=6.25e-09
  YAdder : Sum  OutDataTypeStr=fixdt(1, 32, 19)  SampleTime=6.25e-09
  YSub : Sum  Inputs=+-  OutDataTypeStr=fixdt(1, 32, 19)  AccumDataTypeStr=fixdt(1, 32, 19)  SampleTime=6.25e-09
  ZAdder : Sum  OutDataTypeStr=fixdt(1, 34, 33)  SampleTime=6.25e-09
  ZSub : Sum  Inputs=+-  OutDataTypeStr=fixdt(1, 34, 33)  AccumDataTypeStr=fixdt(1, 34, 33)  SampleTime=6.25e-09
  compare : simulink/Logic and Bit Operations/Compare To Constant  relop=<  const=double(0)  OutDataTypeStr=boolean
  dynamic_shift : ArithShift  BitShiftNumberSource=Input port  BitShiftDirection=Right
      settings: InputPortMap=u0,p1
  dynamic_shift1 : ArithShift  BitShiftNumberSource=Input port  BitShiftDirection=Right
      settings: InputPortMap=u0,p1
  rd_{0..9} (10 alike) : Delay  DelayLength=double(1)  InitialCondition=0  SampleTime=6.25e-09
  xout : Outport  OutDataTypeStr=fixdt(1, 32, 19)  SampleTime=6.25e-09
  yout : Outport  Port=2  OutDataTypeStr=fixdt(1, 32, 19)  SampleTime=6.25e-09
  zout : Outport  Port=3  OutDataTypeStr=fixdt(1, 34, 33)  SampleTime=6.25e-09
  wires:
  MuxX/1 -> xout/1
  rd_2/1 -> MuxX/1
  rd_6/1 -> MuxY/3
  rd_3/1 -> MuxX/2, MuxZ/2, MuxY/2
  rd_5/1 -> MuxY/1
  rd_9/1 -> MuxZ/3
  XSubtractor/1 -> rd_2/1
  YSub/1 -> rd_6/1
  YAdder/1 -> rd_5/1
  yin/1 -> rd_1/1
  xin/1 -> rd_0/1
  MuxY/1 -> yout/1
  zin/1 -> rd_7/1
  rd_4/1 -> MuxX/3
  rd_0/1 -> dynamic_shift/1, XSubtractor/1, XAdder/1
  rd_8/1 -> MuxZ/1
  rd_1/1 -> compare/1, dynamic_shift1/1, YAdder/1, YSub/1
  lut_value/1 -> ZSub/2, ZAdder/2
  MuxZ/1 -> zout/1
  rd_7/1 -> ZSub/1, ZAdder/1
  idx/1 -> dynamic_shift/2, dynamic_shift1/2
  ZAdder/1 -> rd_9/1
  compare/1 -> rd_3/1
  dynamic_shift/1 -> YAdder/2, YSub/2
  dynamic_shift1/1 -> XSubtractor/2, XAdder/2
  XAdder/1 -> rd_4/1
  ZSub/1 -> rd_8/1

== system gm_wlanhdlTimeAndFrequencySynchronization/WLANTimeAndFrequencySynchronization/Coarse CFO Estimation and Correction/Coarse CFO Estimation/Iteration3 ==
  xin : Inport  OutDataTypeStr=fixdt(1, 32, 19)  SampleTime=6.25e-09
  yin : Inport  Port=2  OutDataTypeStr=fixdt(1, 32, 19)  SampleTime=6.25e-09
  zin : Inport  Port=3  OutDataTypeStr=fixdt(1, 34, 33)  SampleTime=6.25e-09
  lut_value : Inport  Port=4  OutDataTypeStr=fixdt(0, 31, 33)  SampleTime=6.25e-09
  idx : Inport  Port=5  OutDataTypeStr=fixdt(0, 6, 0)  SampleTime=6.25e-09
  MuxX : Switch  Criteria=u2 ~= 0  Threshold="fi(0,0,1,0,\"hex\",\"0\")"  OutDataTypeStr=fixdt(1, 32, 19)  SampleTime=6.25e-09  SaturateOnIntegerOverflow=off  InputSameDT=off
  MuxY : Switch  Criteria=u2 ~= 0  Threshold="fi(0,0,1,0,\"hex\",\"0\")"  OutDataTypeStr=fixdt(1, 32, 19)  SampleTime=6.25e-09  SaturateOnIntegerOverflow=off  InputSameDT=off
  MuxZ : Switch  Criteria=u2 ~= 0  Threshold="fi(0,0,1,0,\"hex\",\"0\")"  OutDataTypeStr=fixdt(1, 34, 33)  SampleTime=6.25e-09  SaturateOnIntegerOverflow=off  InputSameDT=off
  XAdder : Sum  OutDataTypeStr=fixdt(1, 32, 19)  SampleTime=6.25e-09
  XSubtractor : Sum  Inputs=+-  OutDataTypeStr=fixdt(1, 32, 19)  AccumDataTypeStr=fixdt(1, 32, 19)  SampleTime=6.25e-09
  YAdder : Sum  OutDataTypeStr=fixdt(1, 32, 19)  SampleTime=6.25e-09
  YSub : Sum  Inputs=+-  OutDataTypeStr=fixdt(1, 32, 19)  AccumDataTypeStr=fixdt(1, 32, 19)  SampleTime=6.25e-09
  ZAdder : Sum  OutDataTypeStr=fixdt(1, 34, 33)  SampleTime=6.25e-09
  ZSub : Sum  Inputs=+-  OutDataTypeStr=fixdt(1, 34, 33)  AccumDataTypeStr=fixdt(1, 34, 33)  SampleTime=6.25e-09
  compare : simulink/Logic and Bit Operations/Compare To Constant  relop=<  const=double(0)  OutDataTypeStr=boolean
  dynamic_shift : ArithShift  BitShiftNumberSource=Input port  BitShiftDirection=Right
      settings: InputPortMap=u0,p1
  dynamic_shift1 : ArithShift  BitShiftNumberSource=Input port  BitShiftDirection=Right
      settings: InputPortMap=u0,p1
  rd_{0..9} (10 alike) : Delay  DelayLength=double(1)  InitialCondition=0  SampleTime=6.25e-09
  xout : Outport  OutDataTypeStr=fixdt(1, 32, 19)  SampleTime=6.25e-09
  yout : Outport  Port=2  OutDataTypeStr=fixdt(1, 32, 19)  SampleTime=6.25e-09
  zout : Outport  Port=3  OutDataTypeStr=fixdt(1, 34, 33)  SampleTime=6.25e-09
  wires:
  MuxX/1 -> xout/1
  rd_4/1 -> MuxX/3
  rd_2/1 -> MuxX/1
  rd_9/1 -> MuxZ/3
  rd_8/1 -> MuxZ/1
  rd_6/1 -> MuxY/3
  rd_5/1 -> MuxY/1
  XAdder/1 -> rd_4/1
  XSubtractor/1 -> rd_2/1
  MuxZ/1 -> zout/1
  ZSub/1 -> rd_8/1
  yin/1 -> rd_1/1
  rd_3/1 -> MuxX/2, MuxY/2, MuxZ/2
  lut_value/1 -> ZAdder/2, ZSub/2
  rd_1/1 -> compare/1, dynamic_shift1/1, YSub/1, YAdder/1
  compare/1 -> rd_3/1
  idx/1 -> dynamic_shift1/2, dynamic_shift/2
  rd_0/1 -> dynamic_shift/1, XSubtractor/1, XAdder/1
  dynamic_shift/1 -> YSub/2, YAdder/2
  dynamic_shift1/1 -> XAdder/2, XSubtractor/2
  ZAdder/1 -> rd_9/1
  zin/1 -> rd_7/1
  YAdder/1 -> rd_5/1
  MuxY/1 -> yout/1
  xin/1 -> rd_0/1
  rd_7/1 -> ZSub/1, ZAdder/1
  YSub/1 -> rd_6/1

== system gm_wlanhdlTimeAndFrequencySynchronization/WLANTimeAndFrequencySynchronization/Coarse CFO Estimation and Correction/Coarse CFO Estimation/Iteration4 ==
  xin : Inport  OutDataTypeStr=fixdt(1, 32, 19)  SampleTime=6.25e-09
  yin : Inport  Port=2  OutDataTypeStr=fixdt(1, 32, 19)  SampleTime=6.25e-09
  zin : Inport  Port=3  OutDataTypeStr=fixdt(1, 34, 33)  SampleTime=6.25e-09
  lut_value : Inport  Port=4  OutDataTypeStr=fixdt(0, 31, 33)  SampleTime=6.25e-09
  idx : Inport  Port=5  OutDataTypeStr=fixdt(0, 6, 0)  SampleTime=6.25e-09
  MuxX : Switch  Criteria=u2 ~= 0  Threshold="fi(0,0,1,0,\"hex\",\"0\")"  OutDataTypeStr=fixdt(1, 32, 19)  SampleTime=6.25e-09  SaturateOnIntegerOverflow=off  InputSameDT=off
  MuxY : Switch  Criteria=u2 ~= 0  Threshold="fi(0,0,1,0,\"hex\",\"0\")"  OutDataTypeStr=fixdt(1, 32, 19)  SampleTime=6.25e-09  SaturateOnIntegerOverflow=off  InputSameDT=off
  MuxZ : Switch  Criteria=u2 ~= 0  Threshold="fi(0,0,1,0,\"hex\",\"0\")"  OutDataTypeStr=fixdt(1, 34, 33)  SampleTime=6.25e-09  SaturateOnIntegerOverflow=off  InputSameDT=off
  XAdder : Sum  OutDataTypeStr=fixdt(1, 32, 19)  SampleTime=6.25e-09
  XSubtractor : Sum  Inputs=+-  OutDataTypeStr=fixdt(1, 32, 19)  AccumDataTypeStr=fixdt(1, 32, 19)  SampleTime=6.25e-09
  YAdder : Sum  OutDataTypeStr=fixdt(1, 32, 19)  SampleTime=6.25e-09
  YSub : Sum  Inputs=+-  OutDataTypeStr=fixdt(1, 32, 19)  AccumDataTypeStr=fixdt(1, 32, 19)  SampleTime=6.25e-09
  ZAdder : Sum  OutDataTypeStr=fixdt(1, 34, 33)  SampleTime=6.25e-09
  ZSub : Sum  Inputs=+-  OutDataTypeStr=fixdt(1, 34, 33)  AccumDataTypeStr=fixdt(1, 34, 33)  SampleTime=6.25e-09
  compare : simulink/Logic and Bit Operations/Compare To Constant  relop=<  const=double(0)  OutDataTypeStr=boolean
  dynamic_shift : ArithShift  BitShiftNumberSource=Input port  BitShiftDirection=Right
      settings: InputPortMap=u0,p1
  dynamic_shift1 : ArithShift  BitShiftNumberSource=Input port  BitShiftDirection=Right
      settings: InputPortMap=u0,p1
  rd_{0..9} (10 alike) : Delay  DelayLength=double(1)  InitialCondition=0  SampleTime=6.25e-09
  xout : Outport  OutDataTypeStr=fixdt(1, 32, 19)  SampleTime=6.25e-09
  yout : Outport  Port=2  OutDataTypeStr=fixdt(1, 32, 19)  SampleTime=6.25e-09
  zout : Outport  Port=3  OutDataTypeStr=fixdt(1, 34, 33)  SampleTime=6.25e-09
  wires:
  MuxX/1 -> xout/1
  rd_2/1 -> MuxX/1
  rd_3/1 -> MuxX/2, MuxY/2, MuxZ/2
  rd_8/1 -> MuxZ/1
  XAdder/1 -> rd_4/1
  XSubtractor/1 -> rd_2/1
  ZSub/1 -> rd_8/1
  yin/1 -> rd_1/1
  MuxZ/1 -> zout/1
  ZAdder/1 -> rd_9/1
  xin/1 -> rd_0/1
  rd_9/1 -> MuxZ/3
  rd_7/1 -> ZSub/1, ZAdder/1
  YAdder/1 -> rd_5/1
  rd_6/1 -> MuxY/3
  zin/1 -> rd_7/1
  lut_value/1 -> ZSub/2, ZAdder/2
  rd_1/1 -> compare/1, dynamic_shift1/1, YAdder/1, YSub/1
  dynamic_shift1/1 -> XSubtractor/2, XAdder/2
  rd_0/1 -> dynamic_shift/1, XSubtractor/1, XAdder/1
  MuxY/1 -> yout/1
  rd_5/1 -> MuxY/1
  idx/1 -> dynamic_shift/2, dynamic_shift1/2
  compare/1 -> rd_3/1
  dynamic_shift/1 -> YAdder/2, YSub/2
  rd_4/1 -> MuxX/3
  YSub/1 -> rd_6/1

== system gm_wlanhdlTimeAndFrequencySynchronization/WLANTimeAndFrequencySynchronization/Coarse CFO Estimation and Correction/Coarse CFO Estimation/Iteration5 ==
  xin : Inport  OutDataTypeStr=fixdt(1, 32, 19)  SampleTime=6.25e-09
  yin : Inport  Port=2  OutDataTypeStr=fixdt(1, 32, 19)  SampleTime=6.25e-09
  zin : Inport  Port=3  OutDataTypeStr=fixdt(1, 34, 33)  SampleTime=6.25e-09
  lut_value : Inport  Port=4  OutDataTypeStr=fixdt(0, 31, 33)  SampleTime=6.25e-09
  idx : Inport  Port=5  OutDataTypeStr=fixdt(0, 6, 0)  SampleTime=6.25e-09
  MuxX : Switch  Criteria=u2 ~= 0  Threshold="fi(0,0,1,0,\"hex\",\"0\")"  OutDataTypeStr=fixdt(1, 32, 19)  SampleTime=6.25e-09  SaturateOnIntegerOverflow=off  InputSameDT=off
  MuxY : Switch  Criteria=u2 ~= 0  Threshold="fi(0,0,1,0,\"hex\",\"0\")"  OutDataTypeStr=fixdt(1, 32, 19)  SampleTime=6.25e-09  SaturateOnIntegerOverflow=off  InputSameDT=off
  MuxZ : Switch  Criteria=u2 ~= 0  Threshold="fi(0,0,1,0,\"hex\",\"0\")"  OutDataTypeStr=fixdt(1, 34, 33)  SampleTime=6.25e-09  SaturateOnIntegerOverflow=off  InputSameDT=off
  XAdder : Sum  OutDataTypeStr=fixdt(1, 32, 19)  SampleTime=6.25e-09
  XSubtractor : Sum  Inputs=+-  OutDataTypeStr=fixdt(1, 32, 19)  AccumDataTypeStr=fixdt(1, 32, 19)  SampleTime=6.25e-09
  YAdder : Sum  OutDataTypeStr=fixdt(1, 32, 19)  SampleTime=6.25e-09
  YSub : Sum  Inputs=+-  OutDataTypeStr=fixdt(1, 32, 19)  AccumDataTypeStr=fixdt(1, 32, 19)  SampleTime=6.25e-09
  ZAdder : Sum  OutDataTypeStr=fixdt(1, 34, 33)  SampleTime=6.25e-09
  ZSub : Sum  Inputs=+-  OutDataTypeStr=fixdt(1, 34, 33)  AccumDataTypeStr=fixdt(1, 34, 33)  SampleTime=6.25e-09
  compare : simulink/Logic and Bit Operations/Compare To Constant  relop=<  const=double(0)  OutDataTypeStr=boolean
  dynamic_shift : ArithShift  BitShiftNumberSource=Input port  BitShiftDirection=Right
      settings: InputPortMap=u0,p1
  dynamic_shift1 : ArithShift  BitShiftNumberSource=Input port  BitShiftDirection=Right
      settings: InputPortMap=u0,p1
  rd_{0..9} (10 alike) : Delay  DelayLength=double(1)  InitialCondition=0  SampleTime=6.25e-09
  xout : Outport  OutDataTypeStr=fixdt(1, 32, 19)  SampleTime=6.25e-09
  yout : Outport  Port=2  OutDataTypeStr=fixdt(1, 32, 19)  SampleTime=6.25e-09
  zout : Outport  Port=3  OutDataTypeStr=fixdt(1, 34, 33)  SampleTime=6.25e-09
  wires:
  MuxY/1 -> yout/1
  MuxZ/1 -> zout/1
  rd_4/1 -> MuxX/3
  rd_3/1 -> MuxZ/2, MuxX/2, MuxY/2
  rd_8/1 -> MuxZ/1
  XSubtractor/1 -> rd_2/1
  YAdder/1 -> rd_5/1
  yin/1 -> rd_1/1
  rd_9/1 -> MuxZ/3
  zin/1 -> rd_7/1
  compare/1 -> rd_3/1
  rd_0/1 -> dynamic_shift/1, XSubtractor/1, XAdder/1
  rd_5/1 -> MuxY/1
  YSub/1 -> rd_6/1
  idx/1 -> dynamic_shift1/2, dynamic_shift/2
  MuxX/1 -> xout/1
  xin/1 -> rd_0/1
  rd_7/1 -> ZSub/1, ZAdder/1
  rd_6/1 -> MuxY/3
  XAdder/1 -> rd_4/1
  lut_value/1 -> ZAdder/2, ZSub/2
  rd_1/1 -> compare/1, YSub/1, dynamic_shift1/1, YAdder/1
  dynamic_shift/1 -> YSub/2, YAdder/2
  rd_2/1 -> MuxX/1
  ZSub/1 -> rd_8/1
  dynamic_shift1/1 -> XAdder/2, XSubtractor/2
  ZAdder/1 -> rd_9/1

== system gm_wlanhdlTimeAndFrequencySynchronization/WLANTimeAndFrequencySynchronization/Coarse CFO Estimation and Correction/Coarse CFO Estimation/Iteration6 ==
  xin : Inport  OutDataTypeStr=fixdt(1, 32, 19)  SampleTime=6.25e-09
  yin : Inport  Port=2  OutDataTypeStr=fixdt(1, 32, 19)  SampleTime=6.25e-09
  zin : Inport  Port=3  OutDataTypeStr=fixdt(1, 34, 33)  SampleTime=6.25e-09
  lut_value : Inport  Port=4  OutDataTypeStr=fixdt(0, 31, 33)  SampleTime=6.25e-09
  idx : Inport  Port=5  OutDataTypeStr=fixdt(0, 6, 0)  SampleTime=6.25e-09
  MuxX : Switch  Criteria=u2 ~= 0  Threshold="fi(0,0,1,0,\"hex\",\"0\")"  OutDataTypeStr=fixdt(1, 32, 19)  SampleTime=6.25e-09  SaturateOnIntegerOverflow=off  InputSameDT=off
  MuxY : Switch  Criteria=u2 ~= 0  Threshold="fi(0,0,1,0,\"hex\",\"0\")"  OutDataTypeStr=fixdt(1, 32, 19)  SampleTime=6.25e-09  SaturateOnIntegerOverflow=off  InputSameDT=off
  MuxZ : Switch  Criteria=u2 ~= 0  Threshold="fi(0,0,1,0,\"hex\",\"0\")"  OutDataTypeStr=fixdt(1, 34, 33)  SampleTime=6.25e-09  SaturateOnIntegerOverflow=off  InputSameDT=off
  XAdder : Sum  OutDataTypeStr=fixdt(1, 32, 19)  SampleTime=6.25e-09
  XSubtractor : Sum  Inputs=+-  OutDataTypeStr=fixdt(1, 32, 19)  AccumDataTypeStr=fixdt(1, 32, 19)  SampleTime=6.25e-09
  YAdder : Sum  OutDataTypeStr=fixdt(1, 32, 19)  SampleTime=6.25e-09
  YSub : Sum  Inputs=+-  OutDataTypeStr=fixdt(1, 32, 19)  AccumDataTypeStr=fixdt(1, 32, 19)  SampleTime=6.25e-09
  ZAdder : Sum  OutDataTypeStr=fixdt(1, 34, 33)  SampleTime=6.25e-09
  ZSub : Sum  Inputs=+-  OutDataTypeStr=fixdt(1, 34, 33)  AccumDataTypeStr=fixdt(1, 34, 33)  SampleTime=6.25e-09
  compare : simulink/Logic and Bit Operations/Compare To Constant  relop=<  const=double(0)  OutDataTypeStr=boolean
  dynamic_shift : ArithShift  BitShiftNumberSource=Input port  BitShiftDirection=Right
      settings: InputPortMap=u0,p1
  dynamic_shift1 : ArithShift  BitShiftNumberSource=Input port  BitShiftDirection=Right
      settings: InputPortMap=u0,p1
  rd_{0..9} (10 alike) : Delay  DelayLength=double(1)  InitialCondition=0  SampleTime=6.25e-09
  xout : Outport  OutDataTypeStr=fixdt(1, 32, 19)  SampleTime=6.25e-09
  yout : Outport  Port=2  OutDataTypeStr=fixdt(1, 32, 19)  SampleTime=6.25e-09
  zout : Outport  Port=3  OutDataTypeStr=fixdt(1, 34, 33)  SampleTime=6.25e-09
  wires:
  MuxX/1 -> xout/1
  rd_4/1 -> MuxX/3
  MuxZ/1 -> zout/1
  rd_2/1 -> MuxX/1
  rd_9/1 -> MuxZ/3
  rd_3/1 -> MuxX/2, MuxY/2, MuxZ/2
  rd_8/1 -> MuxZ/1
  rd_5/1 -> MuxY/1
  XAdder/1 -> rd_4/1
  MuxY/1 -> yout/1
  XSubtractor/1 -> rd_2/1
  ZSub/1 -> rd_8/1
  rd_6/1 -> MuxY/3
  yin/1 -> rd_1/1
  compare/1 -> rd_3/1
  xin/1 -> rd_0/1
  rd_1/1 -> compare/1, dynamic_shift1/1, YSub/1, YAdder/1
  zin/1 -> rd_7/1
  dynamic_shift/1 -> YSub/2, YAdder/2
  rd_0/1 -> dynamic_shift/1, XSubtractor/1, XAdder/1
  rd_7/1 -> ZSub/1, ZAdder/1
  YAdder/1 -> rd_5/1
  ZAdder/1 -> rd_9/1
  dynamic_shift1/1 -> XAdder/2, XSubtractor/2
  idx/1 -> dynamic_shift1/2, dynamic_shift/2
  lut_value/1 -> ZAdder/2, ZSub/2
  YSub/1 -> rd_6/1

== system gm_wlanhdlTimeAndFrequencySynchronization/WLANTimeAndFrequencySynchronization/Coarse CFO Estimation and Correction/Coarse CFO Estimation/Iteration7 ==
  xin : Inport  OutDataTypeStr=fixdt(1, 32, 19)  SampleTime=6.25e-09
  yin : Inport  Port=2  OutDataTypeStr=fixdt(1, 32, 19)  SampleTime=6.25e-09
  zin : Inport  Port=3  OutDataTypeStr=fixdt(1, 34, 33)  SampleTime=6.25e-09
  lut_value : Inport  Port=4  OutDataTypeStr=fixdt(0, 31, 33)  SampleTime=6.25e-09
  idx : Inport  Port=5  OutDataTypeStr=fixdt(0, 6, 0)  SampleTime=6.25e-09
  MuxX : Switch  Criteria=u2 ~= 0  Threshold="fi(0,0,1,0,\"hex\",\"0\")"  OutDataTypeStr=fixdt(1, 32, 19)  SampleTime=6.25e-09  SaturateOnIntegerOverflow=off  InputSameDT=off
  MuxY : Switch  Criteria=u2 ~= 0  Threshold="fi(0,0,1,0,\"hex\",\"0\")"  OutDataTypeStr=fixdt(1, 32, 19)  SampleTime=6.25e-09  SaturateOnIntegerOverflow=off  InputSameDT=off
  MuxZ : Switch  Criteria=u2 ~= 0  Threshold="fi(0,0,1,0,\"hex\",\"0\")"  OutDataTypeStr=fixdt(1, 34, 33)  SampleTime=6.25e-09  SaturateOnIntegerOverflow=off  InputSameDT=off
  XAdder : Sum  OutDataTypeStr=fixdt(1, 32, 19)  SampleTime=6.25e-09
  XSubtractor : Sum  Inputs=+-  OutDataTypeStr=fixdt(1, 32, 19)  AccumDataTypeStr=fixdt(1, 32, 19)  SampleTime=6.25e-09
  YAdder : Sum  OutDataTypeStr=fixdt(1, 32, 19)  SampleTime=6.25e-09
  YSub : Sum  Inputs=+-  OutDataTypeStr=fixdt(1, 32, 19)  AccumDataTypeStr=fixdt(1, 32, 19)  SampleTime=6.25e-09
  ZAdder : Sum  OutDataTypeStr=fixdt(1, 34, 33)  SampleTime=6.25e-09
  ZSub : Sum  Inputs=+-  OutDataTypeStr=fixdt(1, 34, 33)  AccumDataTypeStr=fixdt(1, 34, 33)  SampleTime=6.25e-09
  compare : simulink/Logic and Bit Operations/Compare To Constant  relop=<  const=double(0)  OutDataTypeStr=boolean
  dynamic_shift : ArithShift  BitShiftNumberSource=Input port  BitShiftDirection=Right
      settings: InputPortMap=u0,p1
  dynamic_shift1 : ArithShift  BitShiftNumberSource=Input port  BitShiftDirection=Right
      settings: InputPortMap=u0,p1
  rd_{0..9} (10 alike) : Delay  DelayLength=double(1)  InitialCondition=0  SampleTime=6.25e-09
  xout : Outport  OutDataTypeStr=fixdt(1, 32, 19)  SampleTime=6.25e-09
  yout : Outport  Port=2  OutDataTypeStr=fixdt(1, 32, 19)  SampleTime=6.25e-09
  zout : Outport  Port=3  OutDataTypeStr=fixdt(1, 34, 33)  SampleTime=6.25e-09
  wires:
  MuxZ/1 -> zout/1
  MuxY/1 -> yout/1
  rd_4/1 -> MuxX/3
  rd_9/1 -> MuxZ/3
  XAdder/1 -> rd_4/1
  XSubtractor/1 -> rd_2/1
  ZSub/1 -> rd_8/1
  yin/1 -> rd_1/1
  YSub/1 -> rd_6/1
  rd_3/1 -> MuxX/2, MuxY/2, MuxZ/2
  xin/1 -> rd_0/1
  MuxX/1 -> xout/1
  zin/1 -> rd_7/1
  rd_1/1 -> compare/1, dynamic_shift1/1, YAdder/1, YSub/1
  idx/1 -> dynamic_shift/2, dynamic_shift1/2
  rd_7/1 -> ZSub/1, ZAdder/1
  rd_2/1 -> MuxX/1
  ZAdder/1 -> rd_9/1
  dynamic_shift/1 -> YAdder/2, YSub/2
  compare/1 -> rd_3/1
  rd_6/1 -> MuxY/3
  dynamic_shift1/1 -> XSubtractor/2, XAdder/2
  rd_8/1 -> MuxZ/1
  rd_5/1 -> MuxY/1
  lut_value/1 -> ZSub/2, ZAdder/2
  rd_0/1 -> dynamic_shift/1, XSubtractor/1, XAdder/1
  YAdder/1 -> rd_5/1
